simulink model "ECCE_tutorial_demo2_part1_v2"  (R2022a)
settings: Solver=FixedStepAuto  StartTime=0.0  StopTime=3/60  FixedStep=1/12000  RelTol=1e-3
undefined symbols (not defined in the file or in its folder): Fault_Inv, GA_th_2, SW, Vdc1, Vdc2, Vdc3, Vdc4, Vdc5
libraries: spsDCVoltageSourceLib x5, spsFullBridgeConverterLib x5, spsSeriesRLCBranchLib x1, spsAlphaBetaZerotodq0Lib x1, spsMeanLib x1, simulink x1, spsVoltageMeasurementLib x1, spspowerguiLib x1
(part 2 of 2)

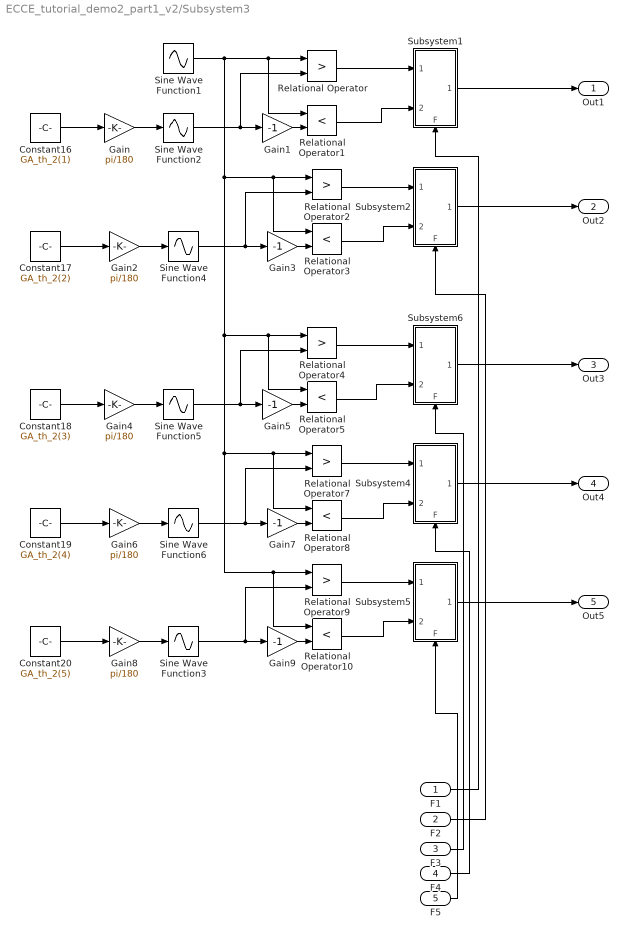
== system ECCE_tutorial_demo2_part1_v2/Subsystem3 ==
  F1 : Inport
  F2 : Inport  Port=2
  F3 : Inport  Port=3
  F4 : Inport  Port=4
  F5 : Inport  Port=5
  Constant16 : Constant  Value=GA_th_2(1)
  Constant17 : Constant  Value=GA_th_2(2)
  Constant18 : Constant  Value=GA_th_2(3)
  Constant19 : Constant  Value=GA_th_2(4)
  Constant20 : Constant  Value=GA_th_2(5)
  Gain{,2,4,6,8} (5 alike) : Gain  Gain=pi/180
  Gain{1,3,5,7,9} (5 alike) : Gain  Gain=-1
  Relational Operator{,2,4,7,9} (5 alike) : RelationalOperator  Operator=>  OutDataTypeStr=boolean  RndMeth=Simplest  InputSameDT=off
  Relational Operator{1,3,5,8,10} (5 alike) : RelationalOperator  Operator=<  OutDataTypeStr=boolean  RndMeth=Simplest  InputSameDT=off
  Sine Wave Function1 : Sin  Frequency=2*pi*60  SampleTime=0
  Sine Wave Function{2..6} (5 alike) : Sin  TimeSource=Use external signal  SampleTime=0
  Subsystem1 : Subsystem
      settings: PortSchema="{\"entries\":[{\"content\":{\"sides\":[{\"content\":{\"connectorIds\":[\"In1\",\"In2\"]},\"type\":\"ConnectorPlacement.EquallySpacedRectSide\",\"uuid\":\"5f14345d-2d5d-483d-90d8-8aa8f8d7da25\"},{\"content\":{\"connectorIds\":[\"Out1\"],\"side\":\"RIGHT\"},\"type\":\"ConnectorPlacement.EquallySpacedRectSide\",\"uuid\":\"3e161696-ca31-43e2-b7bf-a13ac7fb6ba1\"},{\"content\":{\"connectorIds\":[],\"side\":\"TOP\"},\"type\":\"ConnectorPlacement.EquallySpacedRectSide\",\"uuid\":\"8fa02895-2f1e-47bd-8a65-8e37c65d1a87\"},{\"content\":{\"connectorIds\":[\"In3\"],\"side\":\"BOTTOM\"},\"type\":\"ConnectorPlacement.EquallySpacedRectSide\",\"uuid\":\"36cd283d-056f-45a3-b6f0-6bf0daee5395\"}]},\"type\":\"ConnectorPlacement.EquallySpacedConnector\",\"uuid\":\"d0616103-6a76-4dfd-bdc2-221e478031b1\"}],\"packageUris\":[\"http://schema.mathworks.com/mf0/Connector/R2020b\"],\"version\":\"1.0\"}"
  Subsystem2 : Subsystem
      settings: PortSchema="{\"entries\":[{\"content\":{\"sides\":[{\"content\":{\"connectorIds\":[\"In1\",\"In2\"]},\"type\":\"ConnectorPlacement.EquallySpacedRectSide\",\"uuid\":\"5f14345d-2d5d-483d-90d8-8aa8f8d7da25\"},{\"content\":{\"connectorIds\":[\"Out1\"],\"side\":\"RIGHT\"},\"type\":\"ConnectorPlacement.EquallySpacedRectSide\",\"uuid\":\"3e161696-ca31-43e2-b7bf-a13ac7fb6ba1\"},{\"content\":{\"connectorIds\":[],\"side\":\"TOP\"},\"type\":\"ConnectorPlacement.EquallySpacedRectSide\",\"uuid\":\"8fa02895-2f1e-47bd-8a65-8e37c65d1a87\"},{\"content\":{\"connectorIds\":[\"In3\"],\"side\":\"BOTTOM\"},\"type\":\"ConnectorPlacement.EquallySpacedRectSide\",\"uuid\":\"712a4502-34e9-4038-bdd0-4ff6e3ff4ab9\"}]},\"type\":\"ConnectorPlacement.EquallySpacedConnector\",\"uuid\":\"d0616103-6a76-4dfd-bdc2-221e478031b1\"}],\"packageUris\":[\"http://schema.mathworks.com/mf0/Connector/R2020b\"],\"version\":\"1.0\"}"
  Subsystem4 : Subsystem
      settings: PortSchema="{\"entries\":[{\"content\":{\"sides\":[{\"content\":{\"connectorIds\":[\"In1\",\"In2\"]},\"type\":\"ConnectorPlacement.EquallySpacedRectSide\",\"uuid\":\"5f14345d-2d5d-483d-90d8-8aa8f8d7da25\"},{\"content\":{\"connectorIds\":[\"Out1\"],\"side\":\"RIGHT\"},\"type\":\"ConnectorPlacement.EquallySpacedRectSide\",\"uuid\":\"3e161696-ca31-43e2-b7bf-a13ac7fb6ba1\"},{\"content\":{\"connectorIds\":[],\"side\":\"TOP\"},\"type\":\"ConnectorPlacement.EquallySpacedRectSide\",\"uuid\":\"8fa02895-2f1e-47bd-8a65-8e37c65d1a87\"},{\"content\":{\"connectorIds\":[\"In3\"],\"side\":\"BOTTOM\"},\"type\":\"ConnectorPlacement.EquallySpacedRectSide\",\"uuid\":\"86d75a55-3df2-435d-b886-235f200f3608\"}]},\"type\":\"ConnectorPlacement.EquallySpacedConnector\",\"uuid\":\"d0616103-6a76-4dfd-bdc2-221e478031b1\"}],\"packageUris\":[\"http://schema.mathworks.com/mf0/Connector/R2020b\"],\"version\":\"1.0\"}"
  Subsystem5 : Subsystem
      settings: PortSchema="{\"entries\":[{\"content\":{\"sides\":[{\"content\":{\"connectorIds\":[\"In1\",\"In2\"]},\"type\":\"ConnectorPlacement.EquallySpacedRectSide\",\"uuid\":\"5f14345d-2d5d-483d-90d8-8aa8f8d7da25\"},{\"content\":{\"connectorIds\":[\"Out1\"],\"side\":\"RIGHT\"},\"type\":\"ConnectorPlacement.EquallySpacedRectSide\",\"uuid\":\"3e161696-ca31-43e2-b7bf-a13ac7fb6ba1\"},{\"content\":{\"connectorIds\":[],\"side\":\"TOP\"},\"type\":\"ConnectorPlacement.EquallySpacedRectSide\",\"uuid\":\"8fa02895-2f1e-47bd-8a65-8e37c65d1a87\"},{\"content\":{\"connectorIds\":[\"In3\"],\"side\":\"BOTTOM\"},\"type\":\"ConnectorPlacement.EquallySpacedRectSide\",\"uuid\":\"319f308e-a951-488d-98cf-79dcc4f9ddf4\"}]},\"type\":\"ConnectorPlacement.EquallySpacedConnector\",\"uuid\":\"d0616103-6a76-4dfd-bdc2-221e478031b1\"}],\"packageUris\":[\"http://schema.mathworks.com/mf0/Connector/R2020b\"],\"version\":\"1.0\"}"
  Subsystem6 : Subsystem
      settings: PortSchema="{\"entries\":[{\"content\":{\"sides\":[{\"content\":{\"connectorIds\":[\"In1\",\"In2\"]},\"type\":\"ConnectorPlacement.EquallySpacedRectSide\",\"uuid\":\"5f14345d-2d5d-483d-90d8-8aa8f8d7da25\"},{\"content\":{\"connectorIds\":[\"Out1\"],\"side\":\"RIGHT\"},\"type\":\"ConnectorPlacement.EquallySpacedRectSide\",\"uuid\":\"3e161696-ca31-43e2-b7bf-a13ac7fb6ba1\"},{\"content\":{\"connectorIds\":[],\"side\":\"TOP\"},\"type\":\"ConnectorPlacement.EquallySpacedRectSide\",\"uuid\":\"8fa02895-2f1e-47bd-8a65-8e37c65d1a87\"},{\"content\":{\"connectorIds\":[\"In3\"],\"side\":\"BOTTOM\"},\"type\":\"ConnectorPlacement.EquallySpacedRectSide\",\"uuid\":\"dcf360f9-50cf-4544-a649-25291c772c87\"}]},\"type\":\"ConnectorPlacement.EquallySpacedConnector\",\"uuid\":\"d0616103-6a76-4dfd-bdc2-221e478031b1\"}],\"packageUris\":[\"http://schema.mathworks.com/mf0/Connector/R2020b\"],\"version\":\"1.0\"}"
  Out1 : Outport
  Out2 : Outport  Port=2
  Out3 : Outport  Port=3
  Out4 : Outport  Port=4
  Out5 : Outport  Port=5
  wires:
  Gain5/1 -> Relational Operator5/2
  Relational Operator10/1 -> Subsystem5/2(In1)
  Relational Operator4/1 -> Subsystem6/1(In2)
  Sine Wave Function2/1 -> Gain1/1, Relational Operator/2
  Sine Wave Function3/1 -> Relational Operator9/2, Gain9/1
  Gain4/1 -> Sine Wave Function5/1
  Relational Operator/1 -> Subsystem1/1(In2)
  Sine Wave Function4/1 -> Relational Operator2/2, Gain3/1
  Relational Operator9/1 -> Subsystem5/1(In2)
  Gain9/1 -> Relational Operator10/2
  Subsystem5/1(Out1) -> Out5/1
  Gain/1 -> Sine Wave Function2/1
  Sine Wave Function1/1 -> Relational Operator4/1, Relational Operator5/1, Relational Operator9/1, Relational Operator10/1, Relational Operator8/1, Relational Operator7/1, Relational Operator2/1, Relational Operator3/1, Relational Operator1/1, Relational Operator/1
  Gain7/1 -> Relational Operator8/2
  Gain6/1 -> Sine Wave Function6/1
  Sine Wave Function6/1 -> Gain7/1, Relational Operator7/2
  Sine Wave Function5/1 -> Relational Operator4/2, Gain5/1
  Subsystem2/1(Out1) -> Out2/1
  Relational Operator3/1 -> Subsystem2/2(In1)
  Constant20/1 -> Gain8/1
  Subsystem6/1(Out1) -> Out3/1
  F2/1 -> Subsystem2/3(F)
  F1/1 -> Subsystem1/3(F)
  Relational Operator2/1 -> Subsystem2/1(In2)
  Relational Operator1/1 -> Subsystem1/2(In1)
  Constant17/1 -> Gain2/1
  Constant16/1 -> Gain/1
  Gain3/1 -> Relational Operator3/2
  Relational Operator8/1 -> Subsystem4/2(In1)
  Gain1/1 -> Relational Operator1/2
  Gain2/1 -> Sine Wave Function4/1
  Constant19/1 -> Gain6/1
  Relational Operator7/1 -> Subsystem4/1(In2)
  Constant18/1 -> Gain4/1
  Relational Operator5/1 -> Subsystem6/2(In1)
  Gain8/1 -> Sine Wave Function3/1
  Subsystem1/1(Out1) -> Out1/1
  Subsystem4/1(Out1) -> Out4/1
  F4/1 -> Subsystem4/3(F)
  F5/1 -> Subsystem5/3(F)
  F3/1 -> Subsystem6/3(F)

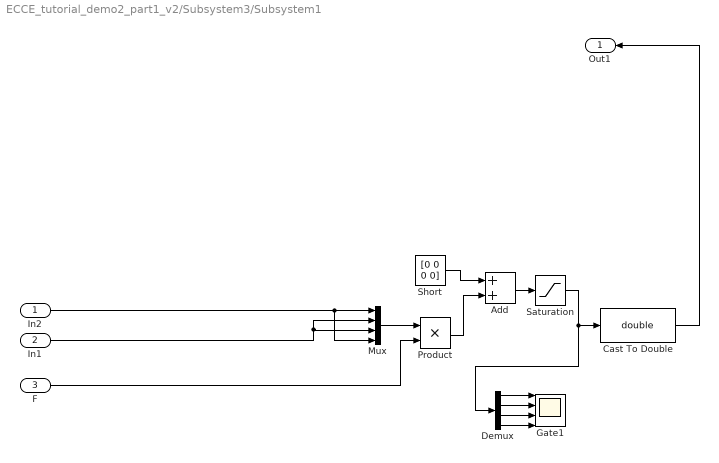
== system ECCE_tutorial_demo2_part1_v2/Subsystem3/Subsystem1 ==
  In2 : Inport
  In1 : Inport  Port=2
  F : Inport  Port=3
  Add : Sum
  Cast To Double : DataTypeConversion  OutDataTypeStr=double  SaturateOnIntegerOverflow=off  RndMeth=Floor
  Demux : Demux
  Gate1 : Scope  NumInputPorts=4
  Mux : Mux
  Product : Product
  Saturation : Saturate  UpperLimit=1  LowerLimit=0
  Short : Constant  Value=[0 0 0 0]
  Out1 : Outport
  wires:
  Mux/1 -> Product/1
  Cast To Double/1 -> Out1/1
  In2/1 -> Mux/4, Mux/1
  In1/1 -> Mux/3, Mux/2
  Product/1 -> Add/2
  Demux/1 -> Gate1/1
  Demux/2 -> Gate1/2
  Demux/3 -> Gate1/3
  Demux/4 -> Gate1/4
  Short/1 -> Add/1
  Add/1 -> Saturation/1
  Saturation/1 -> Demux/1, Cast To Double/1
  F/1 -> Product/2

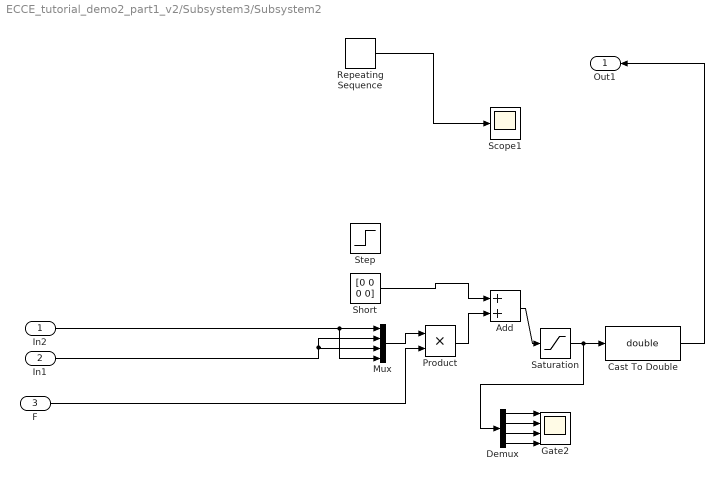
== system ECCE_tutorial_demo2_part1_v2/Subsystem3/Subsystem2 ==
  In2 : Inport
  In1 : Inport  Port=2
  F : Inport  Port=3
  Add : Sum
  Cast To Double : DataTypeConversion  OutDataTypeStr=double  SaturateOnIntegerOverflow=off  RndMeth=Floor
  Demux : Demux
  Gate2 : Scope  NumInputPorts=4
  Mux : Mux
  Product : Product
  Repeating Sequence : simulink/Sources/Repeating Sequence  rep_seq_t="[0  3/60 3.01/60 20/60 20.01/60 30/60 ]"  rep_seq_y="[1 1  1 1 1 1 ]"
  Saturation : Saturate  UpperLimit=1  LowerLimit=0
  Scope1 : Scope
  Short : Constant  Value=[0 0 0 0]
  Step : Step  Time=10/60  SampleTime=0
  Out1 : Outport
  wires:
  Repeating Sequence/1 -> Scope1/1
  Short/1 -> Add/1
  Saturation/1 -> Cast To Double/1, Demux/1
  Add/1 -> Saturation/1
  Demux/4 -> Gate2/4
  Demux/3 -> Gate2/3
  Demux/2 -> Gate2/2
  Demux/1 -> Gate2/1
  Product/1 -> Add/2
  In1/1 -> Mux/2, Mux/3
  In2/1 -> Mux/1, Mux/4
  Cast To Double/1 -> Out1/1
  Mux/1 -> Product/1
  F/1 -> Product/2

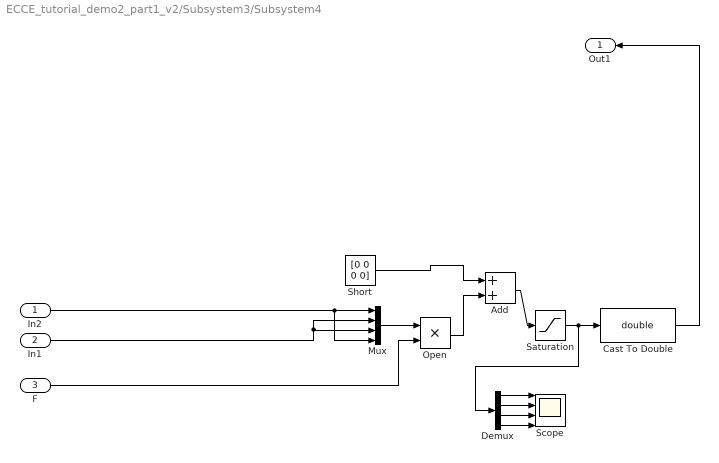
== system ECCE_tutorial_demo2_part1_v2/Subsystem3/Subsystem4 ==
  In2 : Inport
  In1 : Inport  Port=2
  F : Inport  Port=3
  Add : Sum
  Cast To Double : DataTypeConversion  OutDataTypeStr=double  SaturateOnIntegerOverflow=off  RndMeth=Floor
  Demux : Demux
  Mux : Mux
  Open : Product
  Saturation : Saturate  UpperLimit=1  LowerLimit=0
  Scope : Scope  NumInputPorts=4
  Short : Constant  Value=[0 0 0 0]
  Out1 : Outport
  wires:
  Short/1 -> Add/1
  Saturation/1 -> Cast To Double/1, Demux/1
  Add/1 -> Saturation/1
  Demux/4 -> Scope/4
  Demux/3 -> Scope/3
  Demux/2 -> Scope/2
  Demux/1 -> Scope/1
  Open/1 -> Add/2
  In1/1 -> Mux/2, Mux/3
  In2/1 -> Mux/1, Mux/4
  Cast To Double/1 -> Out1/1
  Mux/1 -> Open/1
  F/1 -> Open/2

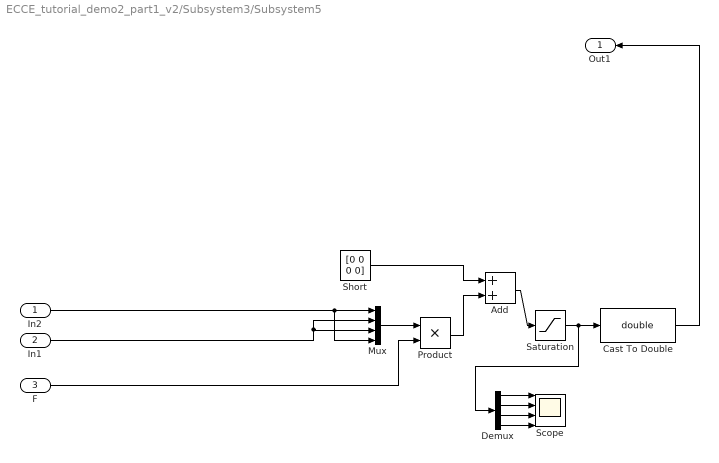
== system ECCE_tutorial_demo2_part1_v2/Subsystem3/Subsystem5 ==
  In2 : Inport
  In1 : Inport  Port=2
  F : Inport  Port=3
  Add : Sum
  Cast To Double : DataTypeConversion  OutDataTypeStr=double  SaturateOnIntegerOverflow=off  RndMeth=Floor
  Demux : Demux
  Mux : Mux
  Product : Product
  Saturation : Saturate  UpperLimit=1  LowerLimit=0
  Scope : Scope  NumInputPorts=4
  Short : Constant  Value=[0 0 0 0]
  Out1 : Outport
  wires:
  Mux/1 -> Product/1
  Cast To Double/1 -> Out1/1
  In2/1 -> Mux/4, Mux/1
  In1/1 -> Mux/3, Mux/2
  Product/1 -> Add/2
  Demux/1 -> Scope/1
  Demux/2 -> Scope/2
  Demux/3 -> Scope/3
  Demux/4 -> Scope/4
  Add/1 -> Saturation/1
  Saturation/1 -> Demux/1, Cast To Double/1
  Short/1 -> Add/1
  F/1 -> Product/2

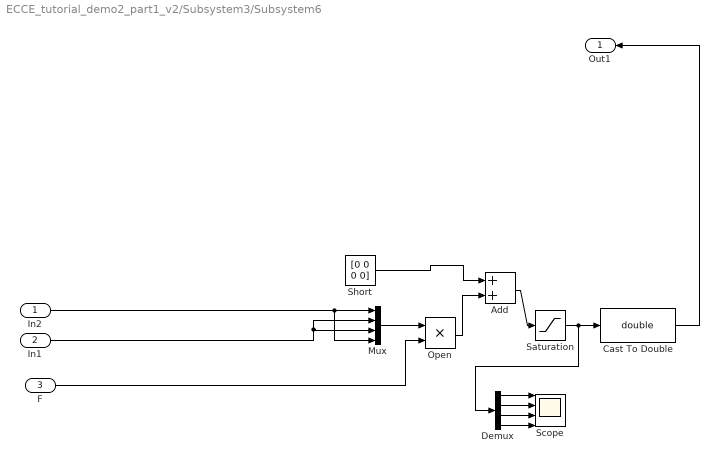
== system ECCE_tutorial_demo2_part1_v2/Subsystem3/Subsystem6 ==
  In2 : Inport
  In1 : Inport  Port=2
  F : Inport  Port=3
  Add : Sum
  Cast To Double : DataTypeConversion  OutDataTypeStr=double  SaturateOnIntegerOverflow=off  RndMeth=Floor
  Demux : Demux
  Mux : Mux
  Open : Product
  Saturation : Saturate  UpperLimit=1  LowerLimit=0
  Scope : Scope  NumInputPorts=4
  Short : Constant  Value=[0 0 0 0]
  Out1 : Outport
  wires:
  Mux/1 -> Open/1
  Cast To Double/1 -> Out1/1
  In2/1 -> Mux/4, Mux/1
  In1/1 -> Mux/3, Mux/2
  Open/1 -> Add/2
  Demux/1 -> Scope/1
  Demux/2 -> Scope/2
  Demux/3 -> Scope/3
  Demux/4 -> Scope/4
  Add/1 -> Saturation/1
  Saturation/1 -> Demux/1, Cast To Double/1
  Short/1 -> Add/1
  F/1 -> Open/2

== matlab function ECCE_tutorial_demo2_part1_v2/Inverter Gate Signal Fault Generator ==
  data: Inv input; G_Inv1 output; G_Inv2 output; G_Inv3 output; G_Inv4 output; G_Inv5 output; SW input
function [G_Inv1,G_Inv2,G_Inv3, G_Inv4,G_Inv5]= fcn(Inv,SW)
    G_Inv1 = [1 1 1 1]; 
    G_Inv2 = [1 1 1 1]; 
    G_Inv3 = [1 1 1 1]; 
    G_Inv4 = [1 1 1 1]; 
    G_Inv5 = [1 1 1 1]; 

    if (Inv==1) && (SW ~= 0)
        G_Inv1(SW) = 0;
    end
    if Inv==2 && (SW ~= 0)
        G_Inv2(SW) = 0;
    end
    if Inv==3 && (SW ~= 0)
        G_Inv3(SW) = 0;
    end
    if Inv==4 && (SW ~= 0)
        G_Inv4(SW) = 0;
    end
    if Inv==5 && (SW ~= 0)
        G_Inv5(SW) = 0;
    end

end
